simulink model "ESP_RTW"  (Simulink 8.7)
settings: Solver=ode1  SolverMode=SingleTasking  StartTime=0.0  StopTime=inf  FixedStep=0.001  RelTol=1e-3
PreLoadFcn:
  | vehicle = 'Car'; if ~length(which('cmcmd')), cmenv; end
  | ESP_RTW_bus
  | ESP_RTW_params
InitFcn:
  | vehicle = 'Car'; if ~length(which('cmcmd')), cmenv; end
  | ESP_RTW_bus
  | ESP_RTW_params
undefined symbols (not defined in the file or in its folder): Area_Front, Area_Rear, ay_max_off, ay_max_on, ay_per_mu_max_off, ay_per_mu_max_on, Brake_ratio, brake_valve_ctrl_kP, cat1mode1_higher, cat1mode1_lower, cat1mode2_higher, cat1mode2_lower, cat1mode3_higher, cat1mode3_lower, cat2mode1_higher, cat2mode1_lower, cat2mode2_higher, cat2mode2_lower, cat2mode3_higher, cat2mode3_lower, delta_vel, diff_lock_fac, diff_lock_off, diff_lock_on, ESP_ctrl_kD, ESP_ctrl_kI, ESP_ctrl_kP, ESP_ctrl_restore_kI, ESP_min_throttle_fac, f_ax, f_slip, g, higherlimit_highvel, higherlimit_lowvel, highervel_fac, highervelocity_fac, InitialConditionForIntegrator, limit_acc, limit_selectlow, limit_starting, limit_vdiff, locktime_throttle, lowerlimit_highvel, lowerlimit_lowvel, lowervel_fac, lowervelocity_fac, min_throttle, MPS2KMPH, MSR_ctrl_kD, MSR_ctrl_kI, MSR_ctrl_kP, MSR_min_throttle_fac, PID_kD_sideslip, PID_kD_yawrate, PID_kI_sideslip, PID_kI_yawrate, PID_kP_sideslip, PID_kP_yawrate, RADpS2RpM, rBrake ... (+37)
libraries: CarMaker4SL x133, simulink x47, simulink_extras x6
(part 4 of 4)

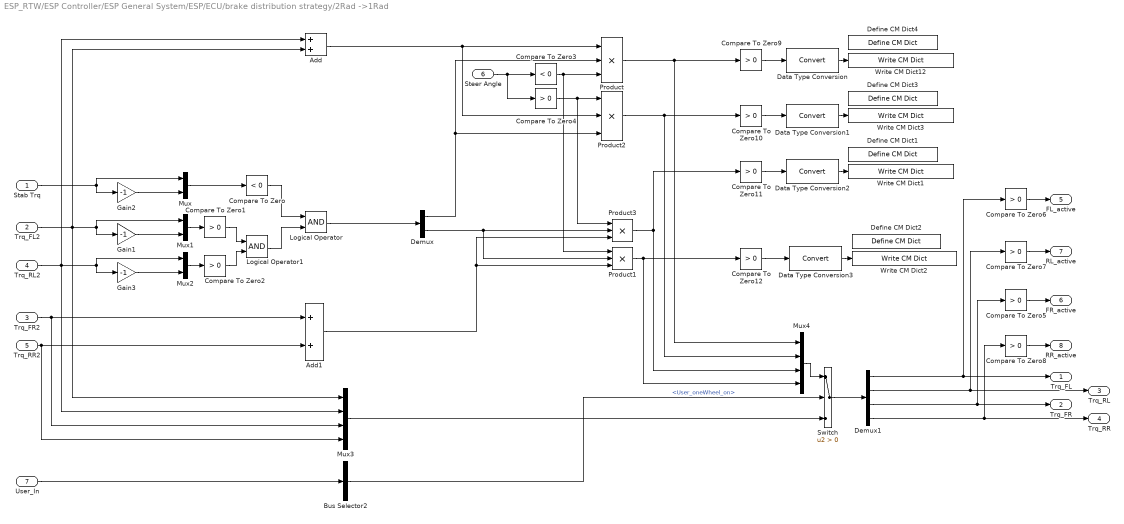
== system ESP_RTW/ESP Controller/ESP General System/ESP/ECU/brake distribution strategy/2Rad ->1Rad ==
  Stab Trq : Inport
  Trq_FL2 : Inport  Port=2
  Trq_FR2 : Inport  Port=3
  Trq_RL2 : Inport  Port=4
  Trq_RR2 : Inport  Port=5
  Steer Angle : Inport  Port=6
  User_In : Inport  Port=7
  Add : Sum
  Add1 : Sum
  Bus Selector2 : BusSelector  OutputSignals=User_oneWheel_on
  Compare To Zero : simulink/Logic and Bit Operations/Compare To Zero  relop=<  OutDataTypeStr=uint8
  Compare To Zero{1..2,4..12} (11 alike) : simulink/Logic and Bit Operations/Compare To Zero  relop=>  OutDataTypeStr=uint8
  Compare To Zero3 : simulink/Logic and Bit Operations/Compare To Zero  relop=<  OutDataTypeStr=uint8
  Data Type Conversion{,1..3} (4 alike) : DataTypeConversion
  Define CM Dict1 : CarMaker4SL/Define CM Dict  xname=ESP.FR_active  xmono=off  xtype=Char  xdvaplace=VC  xnstates=2  xfirststate=0  xinitial=0
  Define CM Dict2 : CarMaker4SL/Define CM Dict  xname=ESP.RR_active  xmono=off  xtype=Char  xdvaplace=VC  xnstates=2  xfirststate=0  xinitial=0
  Define CM Dict3 : CarMaker4SL/Define CM Dict  xname=ESP.RL_active  xmono=off  xtype=Char  xdvaplace=VC  xnstates=2  xfirststate=0  xinitial=0
  Define CM Dict4 : CarMaker4SL/Define CM Dict  xname=ESP.FL_active  xmono=off  xtype=Char  xdvaplace=VC  xnstates=2  xfirststate=0  xinitial=0
  Demux : Demux  Outputs=2
  Demux1 : Demux
  Gain1 : Gain  Gain=-1
  Gain2 : Gain  Gain=-1
  Gain3 : Gain  Gain=-1
  Logical Operator : Logic  AllPortsSameDT=off
  Logical Operator1 : Logic  AllPortsSameDT=off  OutDataTypeStr=boolean
  Mux : Mux  Inputs=2
  Mux1 : Mux  Inputs=2
  Mux2 : Mux  Inputs=2
  Mux3 : Mux
  Mux4 : Mux
  Product{,1..3} (4 alike) : Product  Inputs=3  RndMeth=Zero
  Switch : Switch  Criteria=u2 > Threshold
  Write CM Dict1 : CarMaker4SL/Write CM Dict  xname=ESP.FR_active  xsync=off
  Write CM Dict12 : CarMaker4SL/Write CM Dict  xname=ESP.FL_active  xsync=off
  Write CM Dict2 : CarMaker4SL/Write CM Dict  xname=ESP.RR_active  xsync=off
  Write CM Dict3 : CarMaker4SL/Write CM Dict  xname=ESP.RL_active  xsync=off
  Trq_FL : Outport
  Trq_FR : Outport  Port=2
  Trq_RL : Outport  Port=3
  Trq_RR : Outport  Port=4
  FL_active : Outport  Port=5
  FR_active : Outport  Port=6
  RL_active : Outport  Port=7
  RR_active : Outport  Port=8
  wires:
  User_In/1 -> Bus Selector2/1
  Compare To Zero12/1 -> Data Type Conversion3/1
  Compare To Zero5/1 -> FR_active/1
  Data Type Conversion3/1 -> Write CM Dict2/1
  Data Type Conversion2/1 -> Write CM Dict1/1
  Compare To Zero11/1 -> Data Type Conversion2/1
  Compare To Zero10/1 -> Data Type Conversion1/1
  Data Type Conversion1/1 -> Write CM Dict3/1
  Compare To Zero9/1 -> Data Type Conversion/1
  Bus Selector2/1 -> Switch/2  "<User_oneWheel_on>"
  Demux1/4 -> Compare To Zero8/1, Trq_RR/1
  Demux1/3 -> Compare To Zero5/1, Trq_FR/1
  Demux1/2 -> Compare To Zero7/1, Trq_RL/1
  Demux1/1 -> Compare To Zero6/1, Trq_FL/1
  Switch/1 -> Demux1/1
  Mux4/1 -> Switch/1
  Mux3/1 -> Switch/3
  Data Type Conversion/1 -> Write CM Dict12/1
  Compare To Zero8/1 -> RR_active/1
  Compare To Zero7/1 -> RL_active/1
  Compare To Zero6/1 -> FL_active/1
  Product1/1 -> Compare To Zero12/1, Mux4/4
  Compare To Zero4/1 -> Product3/1, Product2/1
  Product2/1 -> Compare To Zero10/1, Mux4/2
  Compare To Zero3/1 -> Product1/1, Product/3
  Steer Angle/1 -> Compare To Zero4/1, Compare To Zero3/1
  Trq_RR2/1 -> Mux3/4, Add1/2
  Trq_FR2/1 -> Mux3/3, Add1/1
  Product3/1 -> Compare To Zero11/1, Mux4/3
  Demux/2 -> Product1/2, Product3/2
  Add1/1 -> Product1/3, Product3/3
  Product/1 -> Compare To Zero9/1, Mux4/1
  Demux/1 -> Product2/3, Product/2
  Add/1 -> Product2/2, Product/1
  Mux1/1 -> Compare To Zero1/1
  Mux2/1 -> Compare To Zero2/1
  Gain3/1 -> Mux2/2
  Trq_RL2/1 -> Mux3/2, Add/1, Mux2/1, Gain3/1
  Gain1/1 -> Mux1/2
  Trq_FL2/1 -> Mux3/1, Add/2, Mux1/1, Gain1/1
  Mux/1 -> Compare To Zero/1
  Gain2/1 -> Mux/2
  Stab Trq/1 -> Mux/1, Gain2/1
  Compare To Zero2/1 -> Logical Operator1/2
  Compare To Zero1/1 -> Logical Operator1/1
  Logical Operator/1 -> Demux/1
  Logical Operator1/1 -> Logical Operator/2
  Compare To Zero/1 -> Logical Operator/1

== system ESP_RTW/ESP Controller/ESP General System/ESP/helpsignals estimator/mue estimator/estimator_RL ==
  Trq2W_RL : Inport
  Fz_RL : Inport  Port=2
  LongSlip_RL : Inport  Port=3
  Car_vx : Inport  Port=4
  YawRate : Inport  Port=5
  Radius_RL : Inport  Port=6
  " " : simulink/Logic and Bit Operations/Compare To Constant  relop=>=  const=v_min/3.6  OutDataTypeStr=uint8
  "  " : simulink/Logic and Bit Operations/Compare To Constant  relop=>=  const=0.08  OutDataTypeStr=uint8
  "   " : simulink/Logic and Bit Operations/Compare To Constant  relop=<  const=0.2  OutDataTypeStr=uint8
  "    " : simulink/Logic and Bit Operations/Compare To Constant  relop=<=  const=0.15  OutDataTypeStr=uint8
  Abs : Abs
  Compare To Constant2 : simulink/Logic and Bit Operations/Compare To Constant  relop=>  const=-0.05  OutDataTypeStr=uint8
  Compare To Zero : simulink/Logic and Bit Operations/Compare To Zero  relop=>  OutDataTypeStr=uint8
  Compare To Zero1 : simulink/Logic and Bit Operations/Compare To Zero  relop=<  OutDataTypeStr=uint8
  Compare To Zero2 : simulink/Logic and Bit Operations/Compare To Zero  relop=>  OutDataTypeStr=uint8
  Compare To Zero3 : simulink/Logic and Bit Operations/Compare To Zero  relop=>  OutDataTypeStr=uint8
  Constant : Constant  Value=0
  Constant1 : Constant
  Divide1 : Product  Inputs=**
  Divide2 : Product  Inputs=*/
  Divide3 : Product  Inputs=*/
  Gain : Gain  Gain=-1
  Gain1 : Gain  Gain=0.5
  Logical Operator : Logic  Inputs=4  AllPortsSameDT=off  OutDataTypeStr=boolean
  Logical Operator1 : Logic  AllPortsSameDT=off  OutDataTypeStr=boolean
  Logical Operator2 : Logic  AllPortsSameDT=off  OutDataTypeStr=boolean
  Lookup Table : Lookup  InputValues=[0.8 1.8 5.2 6.9 9.5]  Table=[0.1 0.2 0.5 0.7 1]  LookUpMeth=Interpolation-Use End Values
  Memory : Memory
  Subtract : Sum  Inputs=+-
  Subtract1 : Sum
  Switch : Switch  Criteria=u2 > Threshold
  Switch1 : Switch  Criteria=u2 > Threshold
  Triggered Subsystem : Subsystem  TreatAsAtomicUnit=on
  Triggered Subsystem1 : Subsystem  TreatAsAtomicUnit=on
  mue_est_RL : Outport
  wires:
  "   "/1 -> Logical Operator/4
  Abs/1 -> "   "/1
  YawRate/1 -> Abs/1
  Switch1/1 -> mue_est_RL/1
  LongSlip_RL/1 -> Gain/1
  Radius_RL/1 -> Divide1/2
  Fz_RL/1 -> Divide1/1
  Trq2W_RL/1 -> Divide2/1
  Gain1/1 -> Switch1/1
  Constant1/1 -> Switch1/3
  Subtract1/1 -> Gain1/1
  Logical Operator2/1 -> Switch1/2
  Compare To Zero3/1 -> Logical Operator2/2
  Compare To Zero2/1 -> Logical Operator2/1
  Triggered Subsystem1/1(Out1) -> Subtract1/2, Compare To Zero3/1
  Triggered Subsystem/1(Out1) -> Compare To Zero2/1, Subtract1/1
  " "/1 -> Logical Operator/3
  Car_vx/1 -> " "/1
  Logical Operator1/1 -> Triggered Subsystem1/Trigger
  Compare To Constant2/1 -> Logical Operator1/2
  Compare To Zero1/1 -> Logical Operator1/1
  Compare To Zero/1 -> Triggered Subsystem/Trigger
  Subtract/1 -> Compare To Zero/1, Compare To Constant2/1, Compare To Zero1/1
  Memory/1 -> Subtract/2
  Lookup Table/1 -> Triggered Subsystem1/1(In1), Triggered Subsystem/1(In1), Subtract/1, Memory/1
  Gain/1 -> "    "/1, "  "/1, Divide3/2
  Constant/1 -> Switch/3
  Switch/1 -> Lookup Table/1
  Divide3/1 -> Switch/1
  Logical Operator/1 -> Switch/2
  "    "/1 -> Logical Operator/2
  "  "/1 -> Logical Operator/1
  Divide2/1 -> Divide3/1
  Divide1/1 -> Divide2/2

== system ESP_RTW/ESP Controller/ESP General System/ESP/helpsignals estimator/mue estimator/estimator_RR ==
  Trq2W_RR : Inport
  Fz_RR : Inport  Port=2
  LongSlip_RR : Inport  Port=3
  Car_vx : Inport  Port=4
  YawRate : Inport  Port=5
  Radius_RR : Inport  Port=6
  " " : simulink/Logic and Bit Operations/Compare To Constant  relop=>=  const=v_min/3.6  OutDataTypeStr=uint8
  "  " : simulink/Logic and Bit Operations/Compare To Constant  relop=>=  const=0.08  OutDataTypeStr=uint8
  "   " : simulink/Logic and Bit Operations/Compare To Constant  relop=<  const=0.2  OutDataTypeStr=uint8
  "    " : simulink/Logic and Bit Operations/Compare To Constant  relop=<=  const=0.15  OutDataTypeStr=uint8
  Abs : Abs
  Compare To Constant2 : simulink/Logic and Bit Operations/Compare To Constant  relop=>  const=-0.05  OutDataTypeStr=uint8
  Compare To Zero : simulink/Logic and Bit Operations/Compare To Zero  relop=>  OutDataTypeStr=uint8
  Compare To Zero1 : simulink/Logic and Bit Operations/Compare To Zero  relop=<  OutDataTypeStr=uint8
  Compare To Zero2 : simulink/Logic and Bit Operations/Compare To Zero  relop=>  OutDataTypeStr=uint8
  Compare To Zero3 : simulink/Logic and Bit Operations/Compare To Zero  relop=>  OutDataTypeStr=uint8
  Constant : Constant  Value=0
  Constant1 : Constant
  Divide1 : Product  Inputs=**
  Divide2 : Product  Inputs=*/
  Divide3 : Product  Inputs=*/
  Gain : Gain  Gain=-1
  Gain1 : Gain  Gain=0.5
  Logical Operator : Logic  Inputs=4  AllPortsSameDT=off  OutDataTypeStr=boolean
  Logical Operator1 : Logic  AllPortsSameDT=off  OutDataTypeStr=boolean
  Logical Operator2 : Logic  AllPortsSameDT=off  OutDataTypeStr=boolean
  Lookup Table : Lookup  InputValues=[0.8 1.8 5.2 6.9 9.5]  Table=[0.1 0.2 0.5 0.7 1]  LookUpMeth=Interpolation-Use End Values
  Memory : Memory
  Subtract : Sum  Inputs=+-
  Subtract1 : Sum
  Switch : Switch  Criteria=u2 > Threshold
  Switch1 : Switch  Criteria=u2 > Threshold
  Triggered Subsystem : Subsystem  TreatAsAtomicUnit=on
  Triggered Subsystem1 : Subsystem  TreatAsAtomicUnit=on
  mue_est_RR : Outport
  wires:
  "   "/1 -> Logical Operator/4
  Abs/1 -> "   "/1
  YawRate/1 -> Abs/1
  Switch1/1 -> mue_est_RR/1
  LongSlip_RR/1 -> Gain/1
  Radius_RR/1 -> Divide1/2
  Fz_RR/1 -> Divide1/1
  Trq2W_RR/1 -> Divide2/1
  Gain1/1 -> Switch1/1
  Constant1/1 -> Switch1/3
  Subtract1/1 -> Gain1/1
  Logical Operator2/1 -> Switch1/2
  Compare To Zero3/1 -> Logical Operator2/2
  Compare To Zero2/1 -> Logical Operator2/1
  Triggered Subsystem1/1(Out1) -> Subtract1/2, Compare To Zero3/1
  Triggered Subsystem/1(Out1) -> Compare To Zero2/1, Subtract1/1
  " "/1 -> Logical Operator/3
  Car_vx/1 -> " "/1
  Logical Operator1/1 -> Triggered Subsystem1/Trigger
  Compare To Constant2/1 -> Logical Operator1/2
  Compare To Zero1/1 -> Logical Operator1/1
  Compare To Zero/1 -> Triggered Subsystem/Trigger
  Subtract/1 -> Compare To Zero/1, Compare To Constant2/1, Compare To Zero1/1
  Memory/1 -> Subtract/2
  Lookup Table/1 -> Triggered Subsystem1/1(In1), Triggered Subsystem/1(In1), Subtract/1, Memory/1
  Gain/1 -> "    "/1, "  "/1, Divide3/2
  Constant/1 -> Switch/3
  Switch/1 -> Lookup Table/1
  Divide3/1 -> Switch/1
  Logical Operator/1 -> Switch/2
  "    "/1 -> Logical Operator/2
  "  "/1 -> Logical Operator/1
  Divide2/1 -> Divide3/1
  Divide1/1 -> Divide2/2

== system ESP_RTW/ESP Controller/ESP General System/ABS/ABS ECU/select_low/ABS_ValveCtrl_rear/Duty ==
  Constant1 : Constant  Value=1/t_Sensor
  Gain : Gain
  Integrator : Integrator  ExternalReset=either
  Pulse Generator : DiscretePulseGenerator  PulseType=Time based  Period=t_Sensor*2  PulseWidth=50
  SZ : Outport
  wires:
  Constant1/1 -> Gain/1
  Pulse Generator/1 -> Integrator/2
  Integrator/1 -> SZ/1
  Gain/1 -> Integrator/1

== system ESP_RTW/ESP Controller/ESP General System/ESP/ECU/Motor management strategy/restoration to driver/I-Controller ==
  u : Inport
  RESET : Inport  Port=2
  I0 : Inport  Port=3
  Integral Gain : Gain  Gain=ESP_ctrl_restore_kI
  Integrator : Integrator  ExternalReset=either  InitialConditionSource=external  InitialCondition=InitialConditionForIntegrator
  y : Outport  InitialOutput=0
  wires:
  I0/1 -> Integrator/3
  u/1 -> Integral Gain/1
  RESET/1 -> Integrator/2
  Integral Gain/1 -> Integrator/1
  Integrator/1 -> y/1

== system ESP_RTW/ESP Controller/ESP General System/ESP/ECU/Motor management strategy/restoration to driver/lock_signal for n s ==
  Start_value : Inport
  " " : simulink/Logic and Bit Operations/Compare To Constant  relop=>  const=0  OutDataTypeStr=uint8
  Constant : Constant  Value=locktime_throttle
  Data Type Conversion : DataTypeConversion
  Integrator : Integrator  ExternalReset=falling
  Logical Operator3 : Logic  AllPortsSameDT=off  OutDataTypeStr=boolean
  Relational Operator : RelationalOperator  Operator=<=  OutDataTypeStr=boolean
  Triggered Subsystem : Subsystem  TreatAsAtomicUnit=on
  Start_value_locked : Outport
  wires:
  Constant/1 -> Relational Operator/2
  Logical Operator3/1 -> Data Type Conversion/1
  Data Type Conversion/1 -> Start_value_locked/1
  Relational Operator/1 -> Logical Operator3/2
  " "/1 -> Logical Operator3/1
  Triggered Subsystem/1(Out1) -> Integrator/1
  Integrator/1 -> Relational Operator/1, " "/1
  Start_value/1 -> Integrator/2, Triggered Subsystem/Trigger

== system ESP_RTW/ESP Controller/ESP General System/ESP/helpsignals estimator/mue estimator/estimator_RL/Triggered Subsystem ==
  In1 : Inport
  Trigger : TriggerPort  VariantControl=Variant
  Out1 : Outport
  wires:
  In1/1 -> Out1/1

== system ESP_RTW/ESP Controller/ESP General System/ESP/helpsignals estimator/mue estimator/estimator_RL/Triggered Subsystem1 ==
  In1 : Inport
  Trigger : TriggerPort  VariantControl=Variant
  Out1 : Outport
  wires:
  In1/1 -> Out1/1

== system ESP_RTW/ESP Controller/ESP General System/ESP/helpsignals estimator/mue estimator/estimator_RR/Triggered Subsystem ==
  In1 : Inport
  Trigger : TriggerPort  VariantControl=Variant
  Out1 : Outport
  wires:
  In1/1 -> Out1/1

== system ESP_RTW/ESP Controller/ESP General System/ESP/helpsignals estimator/mue estimator/estimator_RR/Triggered Subsystem1 ==
  In1 : Inport
  Trigger : TriggerPort  VariantControl=Variant
  Out1 : Outport
  wires:
  In1/1 -> Out1/1

== system ESP_RTW/ESP Controller/ESP General System/ESP/ECU/Motor management strategy/restoration to driver/lock_signal for n s/Triggered Subsystem ==
  Trigger : TriggerPort  TriggerType=falling  VariantControl=Variant
  Constant1 : Constant
  Out1 : Outport  InitialOutput=[0]
  wires:
  Constant1/1 -> Out1/1
